simulink model "bus_system"  (R2022b)
settings: Solver=FixedStepDiscrete  StartTime=0.0  StopTime=T_final  FixedStep=T_sample  RelTol=1e-3
values from neighbouring files (symbols this model uses):
  attack_final_deviations = zeros(n_meas,2)    [run_bus_system.m]
  attack_full_times = attack_start_times + 4    [run_bus_system.m]
  attack_start_times = attack_start_injection*ones(n_meas,1)    [run_bus_system.m]
  C_obsv_d = C_obsv    [run_bus_system.m]
  D_obsv_d = D_obsv    [run_bus_system.m]
  L_obsv = place(A_bar_d.',C_obsv_d.',P).'    [run_bus_system.m]
  load_buses = [zeros(n_gen,1); ones(n_bus-n_gen,1)]    [run_bus_system.m]
  n_bus = size(bus,1)    [run_bus_system.m]
  n_gen = size(gen,1)    [run_bus_system.m]
  x0 = zeros(n_states,1)    [run_bus_system.m]
  x0_hat = x0    [run_bus_system.m]
undefined symbols (not defined in the file or in its folder): A_bar_d, B_bar_d, sigbuilder_block
libraries: simulink x1
settings Model: Creator=oanubi  LastModifiedBy=digitalstorm
settings SolverCC: AlgebraicLoopSolver=TrustRegion
settings DebuggingCC: UnconnectedInputMsg=warning  UnconnectedOutputMsg=warning  UnconnectedLineMsg=warning  SFMachineParentedDataDiag=warning
settings ModelReferenceCC: EnableRefExpFcnMdlSchedulingChecks=on
settings RTWCC: DLArmComputeVersion=19.05

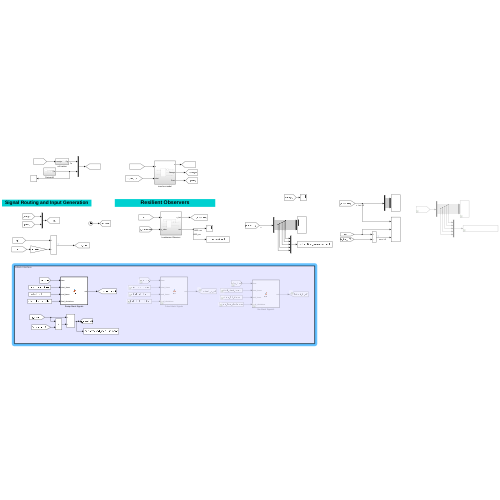
[thumbnail: Simulink's stored preview of the top-level diagram]
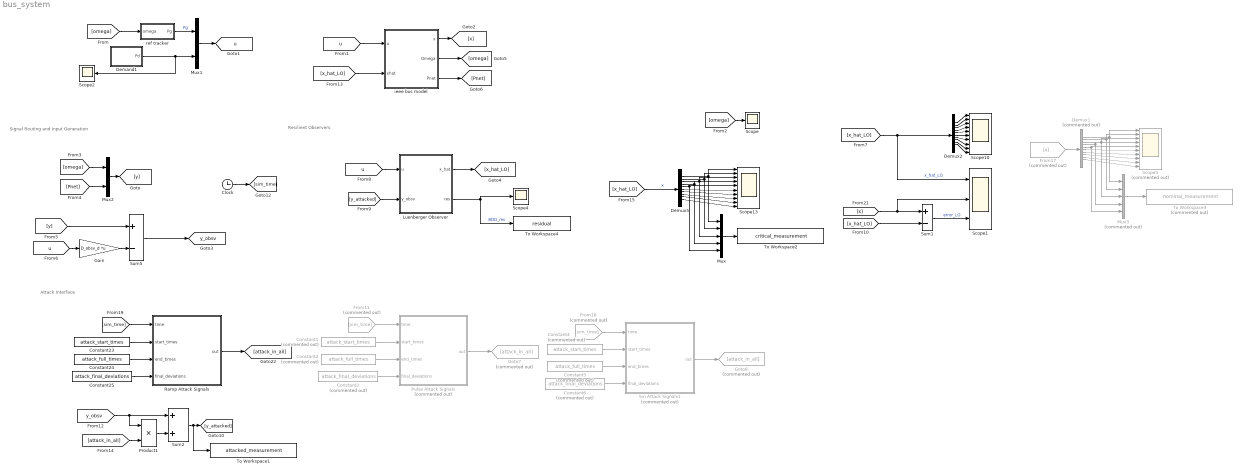
== system bus_system ==
  note: Signal Routing and Input Generation
  note: Resilient Observers
  note: Attack Interface
  Clock : Clock
  Constant1 : Constant  Commented=on  Value=attack_start_times
  Constant2 : Constant  Commented=on  Value=attack_full_times
  Constant23 : Constant  Value=attack_start_times
  Constant24 : Constant  Value=attack_full_times
  Constant25 : Constant  Value=attack_final_deviations
  Constant3 : Constant  Commented=on  Value=attack_final_deviations
  Constant4 : Constant  Commented=on  Value=attack_start_times
  Constant5 : Constant  Commented=on  Value=attack_full_times
  Constant6 : Constant  Commented=on  Value=attack_final_deviations
  Demand1 : Subsystem
  Demux1 : Demux  Commented=on  Outputs=n_states
  Demux2 : Demux  Outputs=n_states
  Demux5 : Demux  Outputs=n_states
  From11 : From  Commented=on  GotoTag=sim_time
  From16 : From  Commented=on  GotoTag=sim_time
  From17 : From  Commented=on  GotoTag=x
  Gain : Gain  Gain=D_obsv_d  Multiplication=Matrix(K*u) (u vector)
  Goto7 : Goto  Commented=on  GotoTag=attack_in_all
  Goto8 : Goto  Commented=on  GotoTag=attack_in_all
  Luenberger Observer : Subsystem
  Mux : Mux  Inputs=5
  Mux1 : Mux  Inputs=2
  Mux2 : Mux  Inputs=2
  Mux3 : Mux  Commented=on  Inputs=5
  Product1 : Product
  Pulse Attack Signals : MATLAB Function  Commented=on  TreatAsAtomicUnit=on
  Ramp Attack Signals : MATLAB Function  TreatAsAtomicUnit=on
  Scope : Scope
  Scope1 : Scope  NumInputPorts=3
  Scope10 : Scope  NumInputPorts=10
  Scope13 : Scope  NumInputPorts=10
  Scope2 : Scope
  Scope3 : Scope  Commented=on  NumInputPorts=10
  Scope4 : Scope
  Sin Attack Signals1 : MATLAB Function  Commented=on  TreatAsAtomicUnit=on
  Sum1 : Sum  Inputs=+-
  Sum2 : Sum
  Sum5 : Sum  Inputs=+-
  To Workspace1 : ToWorkspace  VariableName=attacked_measurement  SaveFormat=Timeseries  SampleTime=-1
  To Workspace2 : ToWorkspace  VariableName=critical_measurement  SaveFormat=Timeseries  SampleTime=-1
  To Workspace3 : ToWorkspace  Commented=on  VariableName=nominal_measurement  SaveFormat=Timeseries  SampleTime=-1
  To Workspace4 : ToWorkspace  VariableName=residual  SaveFormat=Timeseries  SampleTime=-1
  ieee bus model : Subsystem
  ref tracker : Subsystem
  tag scope: u=global, y_obsv=global
  wires:
  Demux5/7 -> Scope13/7
  Gain/1 -> Sum5/2
  Demux2/7 -> Scope10/7
  Demand1/1(Pd) -> Scope2/1, Mux1/2
  ieee bus model/2(Omega) -> [omega]
  Demux5/5 -> Mux/5, Scope13/5
  Demux2/10 -> Scope10/10
  Demux5/2 -> Mux/2, Scope13/2
  [omega] -> ref tracker/1(omega)
  [x] -> Sum1/1, Scope1/2
  Demux5/9 -> Scope13/9
  Demux2/3 -> Scope10/3
  Sum1/1 -> Scope1/3  "error_LO"
  Demux2/5 -> Scope10/5
  Demux2/1 -> Scope10/1
  Demux5/4 -> Mux/4, Scope13/4
  [y] -> Sum5/1
  Mux1/1 -> [u]
  [u] -> ieee bus model/1(u)
  Demux5/6 -> Scope13/6
  [omega] -> Scope/1
  [u] -> Luenberger Observer/1(u)
  ieee bus model/1(x) -> [x]
  [y_attacked] -> Luenberger Observer/2(y_obsv)
  Demux5/3 -> Mux/3, Scope13/3
  Demux2/2 -> Scope10/2
  [x_hat_LO] -> Sum1/2
  Mux2/1 -> [y]
  Demux2/8 -> Scope10/8
  [x_hat_LO] -> Demux2/1, Scope1/1  "x_hat_LO"
  Demux5/8 -> Scope13/8
  Demux2/4 -> Scope10/4
  ref tracker/1(Pg) -> Mux1/1  "Pg"
  [omega] -> Mux2/1
  Demux2/6 -> Scope10/6
  ieee bus model/3(Pnet) -> [Pnet]
  Demux5/10 -> Scope13/10
  Demux5/1 -> Scope13/1, Mux/1
  Demux2/9 -> Scope10/9
  Luenberger Observer/1(x_hat) -> [x_hat_LO]
  [u] -> Gain/1
  [x_hat_LO] -> Demux5/1  "x"
  [Pnet] -> Mux2/2
  [x_hat_LO] -> ieee bus model/2(xhat)
  Product1/1 -> Sum2/2
  [y_obsv] -> Product1/1, Sum2/1
  Constant23/1 -> Ramp Attack Signals/2(start_times)
  Constant25/1 -> Ramp Attack Signals/4(final_deviations)
  [sim_time] -> Ramp Attack Signals/1(time)
  Constant24/1 -> Ramp Attack Signals/3(end_times)
  Ramp Attack Signals/1(out) -> [attack_in_all]
  [attack_in_all] -> Product1/2
  Sum2/1 -> To Workspace1/1, [y_attacked]
  Clock/1 -> [sim_time]
  Mux/1 -> To Workspace2/1
  Sum5/1 -> [y_obsv]
  Mux3/1 -> To Workspace3/1
  Demux1/3 -> Mux3/3, Scope3/3
  Demux1/7 -> Scope3/7
  Demux1/1 -> Scope3/1, Mux3/1
  Demux1/5 -> Mux3/5, Scope3/5
  Demux1/6 -> Scope3/6
  Demux1/4 -> Mux3/4, Scope3/4
  Demux1/10 -> Scope3/10
  Demux1/2 -> Mux3/2, Scope3/2
  Demux1/9 -> Scope3/9
  Demux1/8 -> Scope3/8
  From17/1 -> Demux1/1
  Luenberger Observer/2(res) -> Scope4/1, To Workspace4/1  "BDD_res"
  Constant3/1 -> Pulse Attack Signals/4(final_deviations)
  From11/1 -> Pulse Attack Signals/1(time)
  Pulse Attack Signals/1(out) -> Goto7/1
  Constant1/1 -> Pulse Attack Signals/2(start_times)
  Constant2/1 -> Pulse Attack Signals/3(end_times)
  Constant6/1 -> Sin Attack Signals1/4(final_deviations)
  From16/1 -> Sin Attack Signals1/1(time)
  Sin Attack Signals1/1(out) -> Goto8/1
  Constant4/1 -> Sin Attack Signals1/2(start_times)
  Constant5/1 -> Sin Attack Signals1/3(end_times)

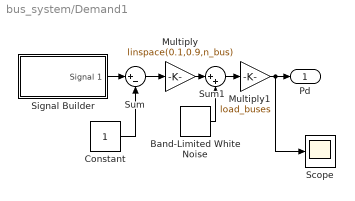
== system bus_system/Demand1 ==
  Band-Limited White Noise : simulink/Sources/Band-Limited White Noise  Cov=1e-8  Ts=0.1  seed=[23341]
  Constant : Constant
  Multiply : Gain  Gain=linspace(0.1,0.9,n_bus)
  Multiply1 : Gain  Gain=load_buses
  Scope : Scope
  Signal Builder : Subsystem  Tag=STV Subsys  LoadFcn=sigbuilder_block('load');  StartFcn=sigbuilder_block('start');  StopFcn=sigbuilder_block('stop');  ClipboardFcn=sigbuilder_block('clipboard');  mask(Sigbuilder block){tuvar=[0:10]}
      mask help: Simulink:masks:SigbuilderBlock_MD
      mask init:
      | if ~strcmp(get_param(bdroot(gcbh),'SimulationStatus'),'stopped') tuvar = sigbuilder_block('maskInit'); end
      settings: CopyFcn=sigbuilder_block('copy');  DeleteFcn=sigbuilder_block('delete');  ModelCloseFcn=sigbuilder_block('modelClose');  PreSaveFcn=sigbuilder_block('preSave');  PauseFcn=sigbuilder_block('pause');  ContinueFcn=sigbuilder_block('continue');  NameChangeFcn=sigbuilder_block('namechange');  OpenFcn=sigbuilder_block('open',[439.2 145.2 550.2 399.9 ]);  CloseFcn=sigbuilder_block('close');
      mask Display: plot(0, 0, 100, 100,[2, 2, 32, 32, 2], [68, 8, 8, 68, 68],[32, 2], [38, 38], [32, 19, 2],[53, 60, 44], [32, 17, 17, 2],[16, 16, 31, 31]);txt = getActiveGroup(gcbh);text(2, 100, txt,'verticalAlignment', 'top');
  Sum : Sum  Inputs=|+-
  Sum1 : Sum  Inputs=|++
  Pd : Outport
  wires:
  Constant/1 -> Sum/2
  Multiply/1 -> Sum1/1
  Band-Limited White Noise/1 -> Sum1/2
  Sum1/1 -> Multiply1/1
  Multiply1/1 -> Scope/1, Pd/1
  Signal Builder/1(Signal 1) -> Sum/1
  Sum/1 -> Multiply/1

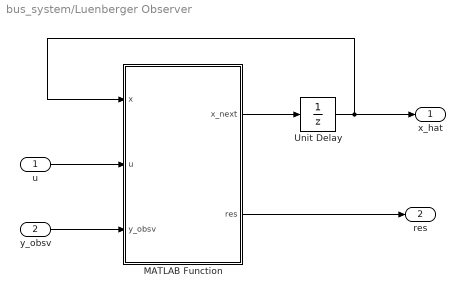
== system bus_system/Luenberger Observer ==
  u : Inport
  y_obsv : Inport  Port=2
  MATLAB Function : MATLAB Function  TreatAsAtomicUnit=on
  Unit Delay : UnitDelay  InitialCondition=x0_hat  SampleTime=-1  HasFrameUpgradeWarning=on
  x_hat : Outport
  res : Outport  Port=2
  wires:
  MATLAB Function/1(x_next) -> Unit Delay/1
  Unit Delay/1 -> x_hat/1, MATLAB Function/1(x)
  u/1 -> MATLAB Function/2(u)
  y_obsv/1 -> MATLAB Function/3(y_obsv)
  MATLAB Function/2(res) -> res/1

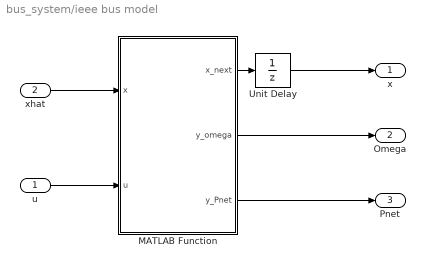
== system bus_system/ieee bus model ==
  u : Inport
  xhat : Inport  Port=2
  MATLAB Function : MATLAB Function  TreatAsAtomicUnit=on
  Unit Delay : UnitDelay  InitialCondition=x0  SampleTime=-1  HasFrameUpgradeWarning=on
  x : Outport
  Omega : Outport  Port=2
  Pnet : Outport  Port=3
  wires:
  MATLAB Function/1(x_next) -> Unit Delay/1
  Unit Delay/1 -> x/1
  u/1 -> MATLAB Function/2(u)
  MATLAB Function/2(y_omega) -> Omega/1
  MATLAB Function/3(y_Pnet) -> Pnet/1
  xhat/1 -> MATLAB Function/1(x)

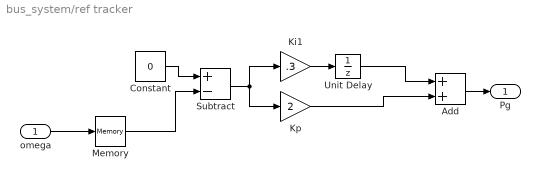
== system bus_system/ref tracker ==
  omega : Inport
  Add : Sum
  Constant : Constant  Value=0
  Ki1 : Gain  Gain=.3
  Kp : Gain  Gain=2
  Memory : Memory  InitialCondition=zeros(n_gen,1)
  Subtract : Sum  Inputs=+-
  Unit Delay : UnitDelay  InitialCondition=zeros(n_gen,1)  SampleTime=-1  HasFrameUpgradeWarning=on
  Pg : Outport
  wires:
  Kp/1 -> Add/2
  Unit Delay/1 -> Add/1
  Add/1 -> Pg/1
  Constant/1 -> Subtract/1
  Subtract/1 -> Ki1/1, Kp/1
  Ki1/1 -> Unit Delay/1
  Memory/1 -> Subtract/2
  omega/1 -> Memory/1

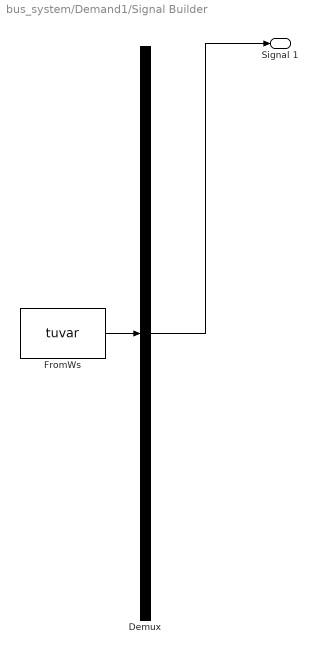
== system bus_system/Demand1/Signal Builder ==
  Demux : Demux  Tag=STV Demux  Outputs=1
      settings: DisplayOption=none
  FromWs : FromWorkspace  Tag=STV FromWs  VariableName=tuvar
      SigBuilderData=|
      | common.afterFinalStr = 'Extrapolate'
      | common.sampleTime = 0
      | dataSet.timeRange = [0 10]
      | dataSet.name = 'Group 1'
      | sbobj.Groups.Name = 'Group 1'
      | sbobj.Groups.Signals.Name = 'Signal 1'
      | sbobj.Groups.Signals.XData = [0 0.46 1.5 2.5 4 5 6 7 10]
      | sbobj.Groups.Signals.YData = [1 1.106 1.2 1.2 0.8 0.8 1 1 1]
  Signal 1 : Outport  Tag=STV Outport
  wires:
  Demux/1 -> Signal 1/1
  FromWs/1 -> Demux/1

== matlab function bus_system/Luenberger Observer/MATLAB Function ==
  data: x_next output; res output; x input; u input; y_obsv input; L_obsv parameter; A_bar_d parameter; C_obsv_d parameter; B_bar_d parameter
function [x_next,res]  = fcn(x,u,y_obsv,L_obsv,A_bar_d,C_obsv_d,B_bar_d)
% Discrete state-space model for system

r = y_obsv - C_obsv_d*x;
x_next = A_bar_d*x + B_bar_d*u + L_obsv*r;

res = norm(r);

== matlab function bus_system/ieee bus model/MATLAB Function ==
  data: x input; x_next output; u input; y_omega output; A_bar_d parameter; C_obsv_d parameter; B_bar_d parameter; D_obsv_d parameter; n_gen parameter; n_bus parameter; y_Pnet output
function [x_next,y_omega,y_Pnet] = fcn(x,u,A_bar_d,C_obsv_d,B_bar_d,D_obsv_d,n_gen, n_bus)
% Discrete state-space model for system

x_next = A_bar_d*x + B_bar_d*u;

y = C_obsv_d*x + D_obsv_d*u;

y_omega = y(1:n_gen);
y_Pnet = y(n_gen+1:n_bus+n_gen);

== matlab function bus_system/Pulse Attack Signals ==
  data: time input; out output; start_times input; end_times input; final_deviations input
function out = fcn(time,start_times,end_times,final_deviations)

delta_times = max(end_times-start_times,0);

deviations = (time<=start_times).*zeros(size(delta_times)) ...
    + ((time>start_times) & (time<=end_times)).*final_deviations ...
    + (time>end_times).*zeros(size(delta_times));

out = deviations;

== matlab function bus_system/Ramp Attack Signals ==
  data: time input; out output; start_times input; end_times input; final_deviations input
function out = fcn(time,start_times,end_times,final_deviations)

delta_times = max(end_times-start_times,0);
ramp_rates  = final_deviations./delta_times;

deviations = (time<=start_times).*zeros(size(delta_times)) ...
    + ((time>start_times) & (time<=end_times)).*(ramp_rates.*(time-start_times)) ...
    + (time>end_times).*(final_deviations);

out = deviations;

== matlab function bus_system/Sin Attack Signals1 ==
  data: time input; out output; start_times input; end_times input; final_deviations input
function out = fcn(time,start_times,end_times,final_deviations)
%% Sin attack
% e = a*sin(b*t)*(start_times < t < end_times)

delta_times = max(end_times-start_times,0);

a = final_deviations(:,1);
b = final_deviations(:,2);
attack_deviation = a.*sin(b.*(time-start_times));

deviations = (time<=start_times).*zeros(size(delta_times)) ...
    + ((time>start_times) & (time<=end_times)).*attack_deviation ...
    + (time>end_times).*zeros(size(delta_times));

out = deviations;
